simulink model "topmodel"  (Simulink 7.7)
settings: Solver=ode45  StartTime=0.0  StopTime=.2  RelTol=1e-3
settings Model: Creator=User  LastModifiedBy=User

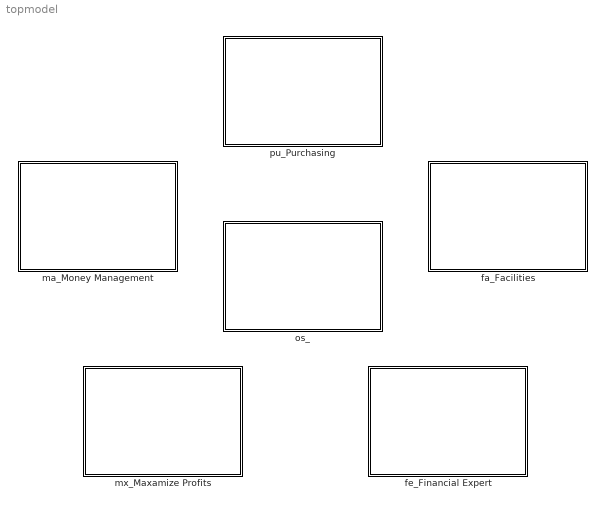
== system topmodel ==
  fa_Facilities : Subsystem
  fe_Financial Expert : Subsystem
  ma_Money Management : Subsystem
  mx_Maxamize Profits : Subsystem
  os_ : Subsystem
  pu_Purchasing : Subsystem

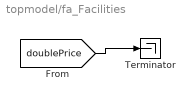
== system topmodel/fa_Facilities ==
  Terminator : Terminator
  wires:
  [doublePrice] -> Terminator/1

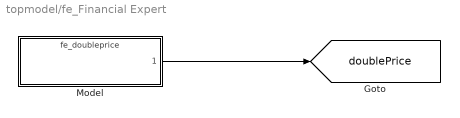
== system topmodel/fe_Financial Expert ==
  Model : ModelReference  ModelNameDialog=fe_doubleprice  SimulationMode=Normal  ModelReferenceVersion=1.5  CopyOfModelName=fe_doubleprice  DefaultDataLogging=on
  tag scope: doublePrice=global
  wires:
  Model/1 -> [doublePrice]

== system topmodel/ma_Money Management ==

== system topmodel/mx_Maxamize Profits ==

== system topmodel/os_ ==

== system topmodel/pu_Purchasing ==
